simulink model "auv_model"  (R2019b)
settings: Solver=VariableStepAuto  StartTime=0.0  StopTime=10.0  RelTol=1e-3
undefined symbols (not defined in the file): m
settings Model: Creator=logan  LastModifiedBy=logan
settings DataIOCC: ReturnWorkspaceOutputs=off
settings DebuggingCC: ArithmeticOperatorsInVariantConditions=warning
settings SFSimCC: CustomCodeUndefinedFunction=UseInterfaceOnly

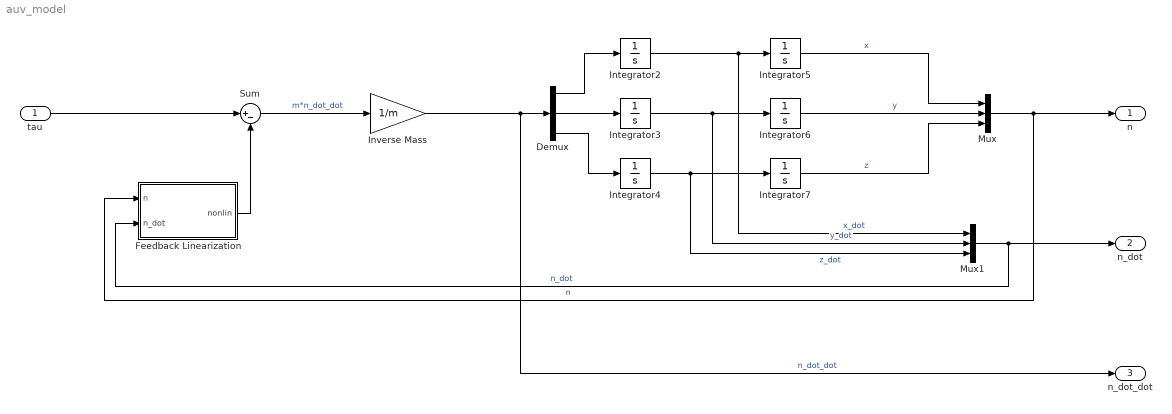
== system auv_model ==
  "tau " : Inport  PortDimensions=3
  Demux : Demux  Outputs=3
  Feedback Linearization : MATLAB Function  TreatAsAtomicUnit=on
  Integrator{2..7} (6 alike) : Integrator
  Inverse Mass : Gain  Gain=1/m
  Mux : Mux  Inputs=3
  Mux1 : Mux  Inputs=3
  Sum : Sum  Inputs=|+-
  n : Outport
  n_dot : Outport  Port=2
  "n_dot_dot " : Outport  Port=3
  wires:
  "tau "/1 -> Sum/1
  Feedback Linearization/1(nonlin) -> Sum/2
  Sum/1 -> Inverse Mass/1  "m*n_dot_dot"
  Inverse Mass/1 -> "n_dot_dot "/1, Demux/1  "n_dot_dot"
  Demux/2 -> Integrator3/1
  Integrator3/1 -> Mux1/2, Integrator6/1  "y_dot"
  Integrator2/1 -> Mux1/1, Integrator5/1  "x_dot"
  Integrator4/1 -> Mux1/3, Integrator7/1  "z_dot"
  Demux/1 -> Integrator2/1
  Demux/3 -> Integrator4/1
  Mux/1 -> Feedback Linearization/1(n), n/1  "n"
  Mux1/1 -> n_dot/1, Feedback Linearization/2(n_dot)  "n_dot"
  Integrator7/1 -> Mux/3  "z"
  Integrator6/1 -> Mux/2  "y"
  Integrator5/1 -> Mux/1  "x"

== matlab function auv_model/Feedback Linearization ==
  data: n input; nonlin output size=3; n_dot input
function nonlin = fcn(n, n_dot)

nonlin = 2*n_dot;
